simulink subsystem "PvtSubSys_VSM_TSR"  (R2020b)
settings: Solver=VariableStepAuto  StartTime=0.0  StopTime=10.0  RelTol=1e-3
values from neighbouring files (symbols this model uses):
  P_VSM_TSR_Dis_keep_SPL_Table : value not decoded    [TSR.sldd]
  P_VSM_TSR_Dis_keep_SPLend = 50.0    [TSR.sldd]
  P_VSM_TSR_Dis_keep_TS_Table : value not decoded    [TSR.sldd]
  P_VSM_TSR_Ena_SPLSupp_Table : value not decoded    [TSR.sldd]
  P_VSM_TSR_Ena_TS_Table : value not decoded    [TSR.sldd]
  P_VSM_TSR_SLIF_Speed_High = 150.0    [TSR.sldd]
  P_VSM_TSR_SLIF_Speed_Low = 0.0    [TSR.sldd]
  P_VSM_TSR_SLW_SnvtySwitch = 0.0    [TSR.sldd]
  P_VSM_TSR_SLW_Speed_Delta_disable = 1.0    [TSR.sldd]
  P_VSM_TSR_SLW_Speed_Delta_enable = 0.0    [TSR.sldd]
  P_VSM_TSR_SLW_Speed_High = 150.0    [TSR.sldd]
  P_VSM_TSR_SLW_Speed_Low = 30.0    [TSR.sldd]
  P_VSM_TSR_SLW_TrafEyeAvtiveDist = 100.0    [TSR.sldd]
  P_VSM_TSR_SLW_Warning_Time = 10.0    [TSR.sldd]
  P_VSM_TSR_SteerWheelAngle = 360.0    [TSR.sldd]
  P_VSM_TSR_SWS_speed_withDir = 9.0    [TSR.sldd]
  P_VSM_TSR_SWS_speed_woDir = 24.0    [TSR.sldd]
libraries: simulink x23
(part 1 of 2)
settings Model: Creator=GW00133806  LastModifiedBy=GW00201299

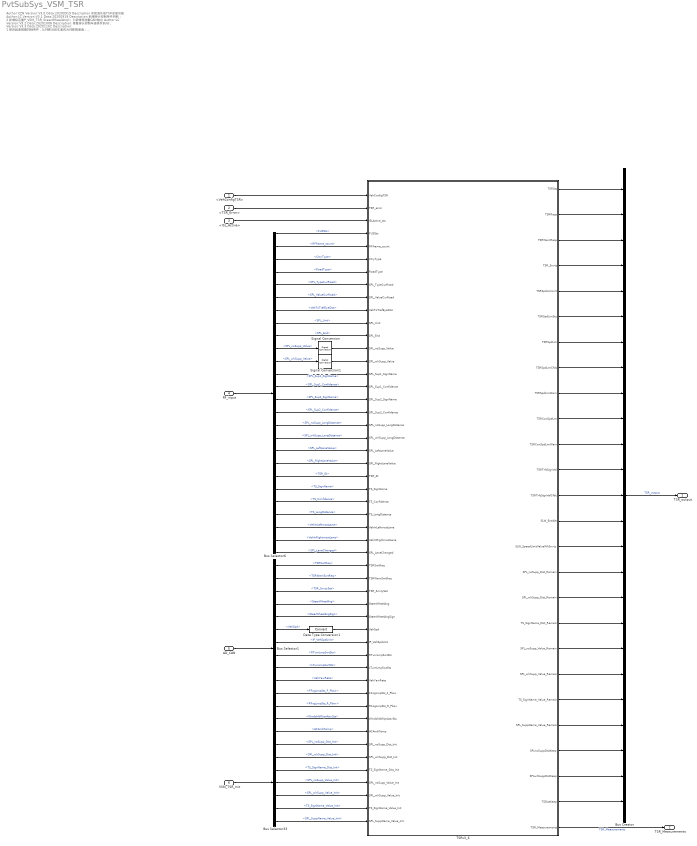
== system PvtSubSys_VSM_TSR ==
  note: Author:CZN
      | Version:V3.0
      | Data:20200919
      | Description:
      | 1.实现海外版TSR全部功能
      | Author:LC
      | Version:V3.1
      | Data:20200919
      | Description:
      | 1.新增掉头抑制条件判断；
      | 2.新增标定量P_VSM_TSR_SteerWheelAngle；
      | 3.新增观测量CAN输出
      | Author:LC
      | Version:V3.2
      | Data:20201008
      | Description:
      | 1.修复掉头抑制车速条件BUG；
      | Version:V3.3
      | Data:20201102
      | Description:
      | 1.修改超速报警抑制条件，从判断当前车速改为判断限速值；
      | 2.修改TSR_error条件下的状态跳转
      | 3.增加了灵敏度设置限幅；
      | 4.更改SLW_Enable信号来源；
      | 5.修复车速单位为英里时，报警值为公里数值问题；
      | 6.更改限速报警限速策略,改为融合发出信息就显示；
      | Version:V3.4
      | Data:20201103
      | Description:
      | 1、新增三个观测量；
      | 2、新增限速使能触发判断；
      | Version:V3.5
      | Data:20201105
      | Description:
      | 1、按照《交通标志信息功能规范》，新增仪表双位灯输出策略；
      | Version:V3.6
      | Data:20201201
      | Description:
      | 1、条件限速使能改为触发式；
      | 20210308
      | 优化转弯限速抑制判断；
      | 20210322
      | 限速条件标志抑制BUG修复；
      | 20210326
      | 1、修复条件限速触发时限速保持距离仍为默认值BUG；
      | 2、修复当超出限速保持距离时，TSR模块将发给仪表的限速清除了，但发给ISL的限速信息漏清BUG；
      | 20210517
      | 修复BUG；当识别到限速标志后3s内不响应解除限速；
      | 20210709:
      | 修复同时识别到限速与接触限速标志后显示解除限速BUG；
  <VehConfigTSR> : Inport
  <TSR_Error> : Inport  Port=2
  <ISL_Active> : Inport  Port=3
  RF_input : Inport  Port=4  OutDataTypeStr=Bus: RFM_TSR_BUS
  AD_CAN : Inport  Port=5  OutDataTypeStr=Bus: AD_TSR_CAN
  VSM_TSR_Init : Inport  Port=6  OutDataTypeStr=Bus: VSM_TSR_INIT_BUS
  Bus Creator : BusCreator  Inputs=25
  Bus Selector1 : BusSelector  OutputSignals=TSRSwtReq,TSRWarnSwtReq,TSR_SnvtySet,SteerWheelAng,SteerWheelAngSign,VehSpd,IP_VehSpdUnit,RTurnLmpSwtSts,LTurnLmpSwtSts,VehYawRate,FFogLmpSts_F_Pbox,RFogLmpSts_R_Pbox,WindshldWiprActvSts,ACAmbTemp
  Bus Selector33 : BusSelector  OutputSignals=SPL_noSupp_Dist_Init,SPL_whSupp_Dist_Init,TS_SignName_Dist_Init,SPL_noSupp_Value_Init,SPL_whSupp_Value_Init,TS_SignName_Value_Init,SPL_SuppName_Value_Init
  Bus Selector6 : BusSelector  OutputSignals=FUSSts,RFframe_count,CtryType,RoadType,SPL_TypeCurRoad,SPL_ValueCurRoad,VehToTrafEyeDist,SPL_Unit,SPL_End,SPL_noSupp_Value,SPL_whSupp_Value,SPL_Sup1_SignName,SPL_Sup1_Confidence,SPL_Sup2_SignName,SPL_Sup2_Confidence,SPL_noSupp_LongDistance,SPL_whSupp_LongDistance,SPL_LeftLaneValue,SPL_RightLaneValue,TSR_ID,TS_SignName,TS_Confidence,TS_LongDistance,VehInLeftmostLane,VehInRightmostLane,SPL_LaneChanged
  Data Type Conversion1 : DataTypeConversion
  Signal Conversion : SignalConversion  OverrideOpt=off
  Signal Conversion1 : SignalConversion  OverrideOpt=off
  TSRv3_6 : Subsystem
  TSR_output : Outport  OutDataTypeStr=Bus: TSR_BUS
  TSR_Measurements : Outport  Port=2  OutDataTypeStr=Bus: VSM_TSR_TSR_Measurements
  wires:
  Signal Conversion/1 -> TSRv3_6/13(SPL_noSupp_Value)
  Bus Selector6/11 -> Signal Conversion1/1  "<SPL_whSupp_Value>"
  Bus Selector33/5 -> TSRv3_6/48(SPL_whSupp_Value_Init)  "<SPL_whSupp_Value_Init>"
  Bus Selector6/26 -> TSRv3_6/29(SPL_LaneChanged)  "<SPL_LaneChanged>"
  Bus Selector1/2 -> TSRv3_6/31(TSRWarnSwtReq)  "<TSRWarnSwtReq>"
  Bus Selector6/16 -> TSRv3_6/19(SPL_noSupp_LongDistance)  "<SPL_noSupp_LongDistance>"
  TSRv3_6/9(TSRSpdLimWarn) -> Bus Creator/9
  Data Type Conversion1/1 -> TSRv3_6/35(VehSpd)
  Bus Selector33/6 -> TSRv3_6/49(TS_SignName_Value_Init)  "<TS_SignName_Value_Init>"
  Bus Selector6/5 -> TSRv3_6/8(SPL_TypeCurRoad)  "<SPL_TypeCurRoad>"
  TSRv3_6/22(SPL_SuppName_Value_Remain) -> Bus Creator/22
  TSRv3_6/1(TSRSts) -> Bus Creator/1
  TSRv3_6/23(SPLnoSuppDistKeep) -> Bus Creator/23
  TSRv3_6/25(TSDistKeep) -> Bus Creator/25
  TSRv3_6/6(TSRSpdLimSts) -> Bus Creator/6
  TSRv3_6/7(TSRSpdLim) -> Bus Creator/7
  Bus Selector33/1 -> TSRv3_6/44(SPL_noSupp_Dist_Init)  "<SPL_noSupp_Dist_Init>"
  Bus Selector6/6 -> TSRv3_6/9(SPL_ValueCurRoad)  "<SPL_ValueCurRoad>"
  Bus Selector6/18 -> TSRv3_6/21(SPL_LeftLaneValue)  "<SPL_LeftLaneValue>"
  Bus Selector6/13 -> TSRv3_6/16(SPL_Sup1_Confidence)  "<SPL_Sup1_Confidence>"
  Bus Selector1/6 -> Data Type Conversion1/1  "<VehSpd>"
  Bus Selector6/24 -> TSRv3_6/27(VehInLeftmostLane)  "<VehInLeftmostLane>"
  TSRv3_6/15(SLW_SpeedLimitValueWhSnvty) -> Bus Creator/15
  TSRv3_6/4(TSR_Snvty) -> Bus Creator/4
  TSRv3_6/10(TSRConSpdLim) -> Bus Creator/10
  TSRv3_6/13(TSRTrfcSignValCfdc) -> Bus Creator/13
  Bus Selector1/11 -> TSRv3_6/40(FFogLmpSts_F_Pbox)  "<FFogLmpSts_F_Pbox>"
  Bus Selector1/8 -> TSRv3_6/37(RTurnLmpSwtSts)  "<RTurnLmpSwtSts>"
  TSRv3_6/26(TSR_Measurements) -> TSR_Measurements/1  "TSR_Measurements"
  TSRv3_6/21(TS_SignName_Value_Remain) -> Bus Creator/21
  Bus Selector6/23 -> TSRv3_6/26(TS_LongDistance)  "<TS_LongDistance>"
  Bus Selector6/22 -> TSRv3_6/25(TS_Confidence)  "<TS_Confidence>"
  Bus Selector6/9 -> TSRv3_6/12(SPL_End)  "<SPL_End>"
  Bus Selector6/14 -> TSRv3_6/17(SPL_Sup2_SignName)  "<SPL_Sup2_SignName>"
  Bus Selector6/8 -> TSRv3_6/11(SPL_Unit)  "<SPL_Unit>"
  Bus Creator/1 -> TSR_output/1  "TSR_output"
  Bus Selector33/4 -> TSRv3_6/47(SPL_noSupp_Value_Init)  "<SPL_noSupp_Value_Init>"
  Bus Selector1/14 -> TSRv3_6/43(ACAmbTemp)  "<ACAmbTemp>"
  Bus Selector1/4 -> TSRv3_6/33(SteerWheelAng)  "<SteerWheelAng>"
  TSRv3_6/24(SPLwhSuppDistKeep) -> Bus Creator/24
  Bus Selector6/2 -> TSRv3_6/5(RFframe_count)  "<RFframe_count>"
  Bus Selector1/10 -> TSRv3_6/39(VehYawRate)  "<VehYawRate>"
  TSRv3_6/14(SLW_Enable) -> Bus Creator/14
  Bus Selector6/1 -> TSRv3_6/4(FUSSts)  "<FUSSts>"
  TSRv3_6/11(TSRConSpdLimWarn) -> Bus Creator/11
  Bus Selector33/2 -> TSRv3_6/45(SPL_whSupp_Dist_Init)  "<SPL_whSupp_Dist_Init>"
  Bus Selector6/4 -> TSRv3_6/7(RoadType)  "<RoadType>"
  TSRv3_6/18(TS_SignName_Dist_Remain) -> Bus Creator/18
  Bus Selector1/3 -> TSRv3_6/32(TSR_SnvtySet)  "<TSR_SnvtySet>"
  TSRv3_6/12(TSRTrfcSignVal) -> Bus Creator/12
  TSRv3_6/19(SPL_noSupp_Value_Remain) -> Bus Creator/19
  Bus Selector1/1 -> TSRv3_6/30(TSRSwtReq)  "<TSRSwtReq>"
  TSRv3_6/8(TSRSpdLimCfdc) -> Bus Creator/8
  Bus Selector6/12 -> TSRv3_6/15(SPL_Sup1_SignName)  "<SPL_Sup1_SignName>"
  TSRv3_6/2(TSRResp) -> Bus Creator/2
  Bus Selector6/21 -> TSRv3_6/24(TS_SignName)  "<TS_SignName>"
  Bus Selector6/19 -> TSRv3_6/22(SPL_RightLaneValue)  "<SPL_RightLaneValue>"
  TSRv3_6/5(TSRSpdLimUnit) -> Bus Creator/5
  Bus Selector6/15 -> TSRv3_6/18(SPL_Sup2_Confidence)  "<SPL_Sup2_Confidence>"
  TSRv3_6/16(SPL_noSupp_Dist_Remain) -> Bus Creator/16
  Bus Selector6/17 -> TSRv3_6/20(SPL_whSupp_LongDistance)  "<SPL_whSupp_LongDistance>"
  Bus Selector1/5 -> TSRv3_6/34(SteerWheelAngSign)  "<SteerWheelAngSign>"
  TSRv3_6/20(SPL_whSupp_Value_Remain) -> Bus Creator/20
  Bus Selector6/10 -> Signal Conversion/1  "<SPL_noSupp_Value>"
  Bus Selector6/3 -> TSRv3_6/6(CtryType)  "<CtryType>"
  Bus Selector33/3 -> TSRv3_6/46(TS_SignName_Dist_Init)  "<TS_SignName_Dist_Init>"
  Bus Selector1/7 -> TSRv3_6/36(IP_VehSpdUnit)  "<IP_VehSpdUnit>"
  <TSR_Error>/1 -> TSRv3_6/2(TSR_error)
  TSRv3_6/17(SPL_whSupp_Dist_Remain) -> Bus Creator/17
  Bus Selector1/12 -> TSRv3_6/41(RFogLmpSts_R_Pbox)  "<RFogLmpSts_R_Pbox>"
  AD_CAN/1 -> Bus Selector1/1
  Bus Selector6/7 -> TSRv3_6/10(VehToTrafEyeDist)  "<VehToTrafEyeDist>"
  Bus Selector1/13 -> TSRv3_6/42(WindshldWiprActvSts)  "<WindshldWiprActvSts>"
  Bus Selector1/9 -> TSRv3_6/38(LTurnLmpSwtSts)  "<LTurnLmpSwtSts>"
  VSM_TSR_Init/1 -> Bus Selector33/1
  RF_input/1 -> Bus Selector6/1
  <ISL_Active>/1 -> TSRv3_6/3(ISLActive_sts)
  Bus Selector6/20 -> TSRv3_6/23(TSR_ID)  "<TSR_ID>"
  Bus Selector33/7 -> TSRv3_6/50(SPL_SuppName_Value_Init)  "<SPL_SuppName_Value_Init>"
  <VehConfigTSR>/1 -> TSRv3_6/1(VehConfigTSR)
  Signal Conversion1/1 -> TSRv3_6/14(SPL_whSupp_Value)
  TSRv3_6/3(TSRWarnResp) -> Bus Creator/3
  Bus Selector6/25 -> TSRv3_6/28(VehInRightmostLane)  "<VehInRightmostLane>"

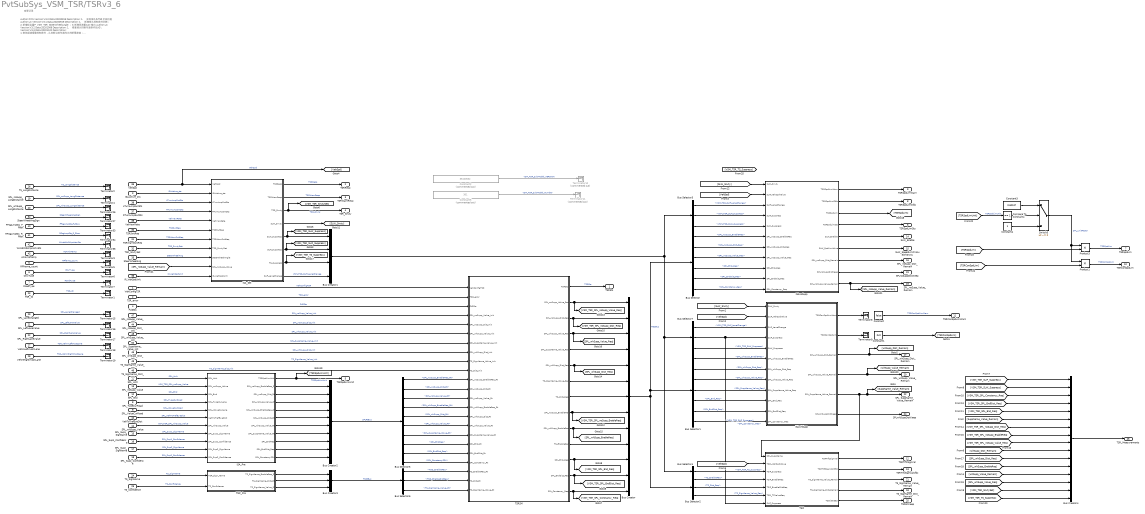
== system PvtSubSys_VSM_TSR/TSRv3_6 ==
  note: 变更记录
  note: Author:CZN
      | Version:V3.0
      | Data:20200919
      | Description:
      | 1.实现海外版TSR全部功能
      | Author:LC
      | Version:V3.1
      | Data:20200919
      | Description:
      | 1.新增掉头抑制条件判断；
      | 2.新增标定量P_VSM_TSR_SteerWheelAngle；
      | 3.新增观测量CAN输出
      | Author:LC
      | Version:V3.2
      | Data:20201008
      | Description:
      | 1.修复掉头抑制车速条件BUG；
      | Version:V3.3
      | Data:20201102
      | Description:
      | 1.修改超速报警抑制条件，从判断当前车速改为判断限速值；
      | 2.修改TSR_error条件下的状态跳转
      | 3.增加了灵敏度设置限幅；
      | 4.更改SLW_Enable信号来源；
      | 5.修复车速单位为英里时，报警值为公里数值问题；
      | 6.更改限速报警限速策略,改为融合发出信息就显示；
      | Version:V3.4
      | Data:20201103
      | Description:
      | 1、新增三个观测量；
      | 2、新增限速使能触发判断；
      | Version:V3.5
      | Data:20201105
      | Description:
      | 1、按照《交通标志信息功能规范》，新增仪表双位灯输出策略；
      | Version:V3.6
      | Data:20201201
      | Description:
      | 1、条件限速使能改为触发式；
      | 20210308
      | 优化转弯限速抑制判断；
      | 20210326
      | 1、修复条件限速触发时限速保持距离仍为默认值BUG；
      | 2、修复当超出限速保持距离时，TSR模块将发给仪表的限速清除了，但发给ISL的限速信息漏清BUG
      | 20210517
      | 修复BUG；当识别到限速标志后3s内不响应解除限速；
  VehConfigTSR : Inport  OutDataTypeStr=uint8
  TSR_error : Inport  Port=2  OutDataTypeStr=uint8
  ISLActive_sts : Inport  Port=3  OutDataTypeStr=boolean
  FUSSts : Inport  Port=4  OutDataTypeStr=uint8
  RFframe_count : Inport  Port=5  OutDataTypeStr=uint32
  CtryType : Inport  Port=6
  RoadType : Inport  Port=7
  SPL_TypeCurRoad : Inport  Port=8  OutDataTypeStr=uint8
  SPL_ValueCurRoad : Inport  Port=9  OutDataTypeStr=uint8
  VehToTrafEyeDist : Inport  Port=10  OutDataTypeStr=uint16
  SPL_Unit : Inport  Port=11  OutDataTypeStr=uint8
  SPL_End : Inport  Port=12  OutDataTypeStr=uint8
  SPL_noSupp_Value : Inport  Port=13  OutDataTypeStr=uint8
  SPL_whSupp_Value : Inport  Port=14  OutDataTypeStr=uint8
  SPL_Sup1_SignName : Inport  Port=15  OutDataTypeStr=uint8
  SPL_Sup1_Confidence : Inport  Port=16  OutDataTypeStr=single
  SPL_Sup2_SignName : Inport  Port=17  OutDataTypeStr=uint8
  SPL_Sup2_Confidence : Inport  Port=18  OutDataTypeStr=single
  SPL_noSupp_LongDistance : Inport  Port=19  OutDataTypeStr=uint8
  SPL_whSupp_LongDistance : Inport  Port=20  OutDataTypeStr=uint8
  SPL_LeftLaneValue : Inport  Port=21  OutDataTypeStr=uint8
  SPL_RightLaneValue : Inport  Port=22  OutDataTypeStr=uint8
  TSR_ID : Inport  Port=23  OutDataTypeStr=uint8
  TS_SignName : Inport  Port=24  OutDataTypeStr=uint8
  TS_Confidence : Inport  Port=25  OutDataTypeStr=single
  TS_LongDistance : Inport  Port=26  OutDataTypeStr=uint8
  VehInLeftmostLane : Inport  Port=27  OutDataTypeStr=uint8
  VehInRightmostLane : Inport  Port=28  OutDataTypeStr=uint8
  SPL_LaneChanged : Inport  Port=29  OutDataTypeStr=uint8
  TSRSwtReq : Inport  Port=30  OutDataTypeStr=boolean
  TSRWarnSwtReq : Inport  Port=31  OutDataTypeStr=boolean
  TSR_SnvtySet : Inport  Port=32  OutDataTypeStr=int8
  SteerWheelAng : Inport  Port=33  OutDataTypeStr=single
  SteerWheelAngSign : Inport  Port=34  OutDataTypeStr=boolean
  VehSpd : Inport  Port=35  OutDataTypeStr=single
  IP_VehSpdUnit : Inport  Port=36  OutDataTypeStr=boolean
  RTurnLmpSwtSts : Inport  Port=37  OutDataTypeStr=boolean
  LTurnLmpSwtSts : Inport  Port=38  OutDataTypeStr=boolean
  VehYawRate : Inport  Port=39  OutDataTypeStr=single
  FFogLmpSts_F_Pbox : Inport  Port=40  OutDataTypeStr=boolean
  RFogLmpSts_R_Pbox : Inport  Port=41  OutDataTypeStr=boolean
  WindshldWiprActvSts : Inport  Port=42  OutDataTypeStr=boolean
  ACAmbTemp : Inport  Port=43  OutDataTypeStr=single
  SPL_noSupp_Dist_Init : Inport  Port=44  OutDataTypeStr=single
  SPL_whSupp_Dist_Init : Inport  Port=45  OutDataTypeStr=single
  TS_SignName_Dist_Init : Inport  Port=46  OutDataTypeStr=single
  SPL_noSupp_Value_Init : Inport  Port=47  OutDataTypeStr=uint8
  SPL_whSupp_Value_Init : Inport  Port=48  OutDataTypeStr=uint8
  TS_SignName_Value_Init : Inport  Port=49  OutDataTypeStr=uint8
  SPL_SuppName_Value_Init : Inport  Port=50  OutDataTypeStr=uint8
  Bus Creator : BusCreator  Inputs=13
  Bus Creator1 : BusCreator  Inputs=4
  Bus Creator2 : BusCreator  Inputs=10
  Bus Creator3 : BusCreator  Inputs=3
  Bus Creator4 : BusCreator  Inputs=16
  Bus Selector : BusSelector  OutputSignals=SPL_noSupp_EnableReq,SPL_noSupp_Dist_Req,SPL_noSupp_Value_Req,SPL_End_Req,SPL_EndDist_Req,SPL_Constancy_Req
  Bus Selector1 : BusSelector  OutputSignals=SPL_whSupp_EnableReq,SPL_whSupp_Dist_Req,SPL_whSupp_Value_Req,SPL_SuppName_Value_Req,SPL_End_Req,SPL_EndDist_Req,SPL_Constancy_Req
  Bus Selector2 : BusSelector  OutputSignals=TS_EnableReq,TS_Dist_Req,TS_SignName_Value_Req
  Bus Selector3 : BusSelector  OutputSignals=VSM_TSR_SLIF_LaneChange,VSM_TSR_SLIF_Suppress,VSM_TSR_SLW_Suppress
  Bus Selector4 : BusSelector  OutputSignals=VSM_TSR_TS_Suppress
  Bus Selector5 : BusSelector  OutputSignals=SPL_noSupp_EnableReq_Rt,SPL_noSupp_Dist_Rt,SPL_noSupp_Value_Rt,SPL_whSupp_EnableReq_Rt,SPL_whSupp_Dist_Rt,SPL_whSupp_Value_Rt,SPL_SuppName_Value_Rt,SPL_EndReq,SPL_EndDist_Req,SPL_ConstancySPL
  Bus Selector6 : BusSelector  OutputSignals=TSD_EnableReq,TSD_EnableDistReq,TS_SignName_Value_Rt
  Bus Selector7 : BusSelector  OutputSignals=VSM_TSR_SLIF_LaneChange,VSM_TSR_SLIF_Suppress,VSM_TSR_SLW_Suppress
  Compare To Constant4 : simulink/Logic and Bit Operations/Compare To Constant  relop===  const=1  OutDataTypeStr=boolean
  Constant : Constant  Value=false  OutDataTypeStr=boolean
  Constant1 : Constant  Value=0x0  OutDataTypeStr=uint8
  Constant2 : Constant  Commented=on  Value=35100532  OutDataTypeStr=uint32
  Constant3 : Constant  Value=0.62137
  Constant4 : Constant
  Constant5 : Constant  Commented=on  Value=301  OutDataTypeStr=uint16
  ISA_Pre : Subsystem
  ISA_Set : Subsystem
  ISAnoSupp : Subsystem
  ISAwhSupp : Subsystem
  Product1 : Product  OutDataTypeStr=uint8
  Product3 : Product  OutDataTypeStr=uint8
  Switch5 : Switch  Criteria=u2 ~= 0  Threshold=1  OutDataTypeStr=single
  TSIF : Subsystem
  TSIF_Pre : Subsystem
  TSRSM : Stateflow chart  TreatAsAtomicUnit=on
  Terminator{1..9,15..19,26..27,33..34,36} (19 alike) : Terminator
  Terminator10 : Terminator  Commented=on
  Terminator11 : Terminator  Commented=on
  TSRSts : Outport
  TSRResp : Outport  Port=2
  TSRWarnResp : Outport  Port=3
  TSR_Snvty : Outport  Port=4  OutDataTypeStr=int8
  TSRSpdLimUnit : Outport  Port=5
  TSRSpdLimSts : Outport  Port=6  OutDataTypeStr=uint8
  TSRSpdLim : Outport  Port=7  OutDataTypeStr=uint8
  TSRSpdLimCfdc : Outport  Port=8  OutDataTypeStr=uint8
  TSRSpdLimWarn : Outport  Port=9  OutDataTypeStr=boolean
  TSRConSpdLim : Outport  Port=10  OutDataTypeStr=uint8
  TSRConSpdLimWarn : Outport  Port=11  OutDataTypeStr=boolean
  TSRTrfcSignVal : Outport  Port=12  OutDataTypeStr=uint8
  TSRTrfcSignValCfdc : Outport  Port=13  OutDataTypeStr=uint8
  SLW_Enable : Outport  Port=14  OutDataTypeStr=boolean
  SLW_SpeedLimitValueWhSnvty : Outport  Port=15  OutDataTypeStr=uint8
  SPL_noSupp_Dist_Remain : Outport  Port=16  OutDataTypeStr=single
  SPL_whSupp_Dist_Remain : Outport  Port=17
  TS_SignName_Dist_Remain : Outport  Port=18  OutDataTypeStr=single
  SPL_noSupp_Value_Remain : Outport  Port=19  OutDataTypeStr=uint8
  SPL_whSupp_Value_Remain : Outport  Port=20  OutDataTypeStr=uint8
  TS_SignName_Value_Remain : Outport  Port=21  OutDataTypeStr=uint8
  SPL_SuppName_Value_Remain : Outport  Port=22  OutDataTypeStr=uint8
  SPLnoSuppDistKeep : Outport  Port=23  OutDataTypeStr=single
  SPLwhSuppDistKeep : Outport  Port=24  OutDataTypeStr=single
  TSDistKeep : Outport  Port=25
  TSR_Measurements : Outport  Port=26
  wires:
  Constant5/1 -> Terminator11/1  "VSM_TSR_SubModel_Number"
  Constant2/1 -> Terminator10/1  "VSM_TSR_SubModel_VERSION"
  ISA_Set/2(TSRWarnResp) -> TSRWarnResp/1  "TSRWarnResp"
  SPL_noSupp_LongDistance/1 -> Terminator4/1  "SPL_noSupp_LongDistance"
  FFogLmpSts_F_Pbox/1 -> Terminator33/1  "FFogLmpSts_F_Pbox"
  ISA_Set/8(SLIF_LaneChange) -> Bus Creator1/4  "VSM_TSR_SLIF_LaneChange"
  ISAnoSupp/3(TSRSpdLim) -> [TSRSpdLim]
  FUSSts/1 -> TSRSM/3(FUSSts)  "FUSSts"
  ISAnoSupp/7(SPL_noSupp_Dist_Remain) -> SPL_noSupp_Dist_Remain/1
  VehConfigTSR/1 -> TSRSM/1(VehConfigTSR)  "VehConfigTSR"
  SPL_noSupp_Value/1 -> ISA_Pre/2(SPL_noSupp_Value)  "VSM_TSR_SPL_noSupp_Value"
  Bus Selector/4 -> ISAnoSupp/9(SPL_End_Req)  "<SPL_End_Req>"
  WindshldWiprActvSts/1 -> Terminator36/1  "WindshldWiprActvSts"
  [VehSpd] -> ISAnoSupp/2(SLIF_VehSpdValue)
  RTurnLmpSwtSts/1 -> ISA_Set/4(RTurnLmpSwtSts)  "RTurnLmpSwtSts"
  ISLActive_sts/1 -> ISA_Set/2(ISLActive_sts)  "ISLActive_sts"
  ISAnoSupp/8(SPLnoSuppDistKeep) -> SPLnoSuppDistKeep/1
  Bus Selector/5 -> ISAnoSupp/10(SPL_EndDist_Req)  "<SPL_EndDist_Req>"
  SPL_ValueCurRoad/1 -> ISA_Pre/5(SPL_ValueCurLane)  "SPL_ValueCurRoad"
  ISA_Set/1(TSRResp) -> TSRResp/1  "TSRResp"
  CtryType/1 -> Terminator6/1  "CtryType"
  TSRWarnSwtReq/1 -> ISA_Set/7(TSRWarnSwtReq)  "TSRWarnSwtReq"
  SteerWheelAngSign/1 -> Terminator27/1  "SteerWheelAngSign"
  VehToTrafEyeDist/1 -> ISA_Pre/6(VehToTrafEyeDist)  "SPL_VehToTrafEyeDist"
  ISA_Set/5(SLW_Suppress) -> Bus Creator1/1, [VSM_TSR_SLW_Suppress]
  TS_SignName/1 -> TSIF_Pre/1(TSR_Sign_Name)  "TS_SignName"
  TSRSwtReq/1 -> ISA_Set/6(TSRSwtReq)  "TSRSwtReq"
  TSIF/3(TS_SignName_Value_Remain) -> TS_SignName_Value_Remain/1
  TSIF/1(TSRTrfcSignVal) -> TSRTrfcSignVal/1
  SPL_whSupp_LongDistance/1 -> Terminator26/1  "SPL_whSupp_LongDistance"
  RFframe_count/1 -> Terminator5/1  "RFframe_count"
  SPL_End/1 -> ISA_Pre/3(SPL_End)  "SPL_End"
  TSRSM/1(TSRSts) -> TSRSts/1  "TSRSts"
  ISAwhSupp/5(SPL_SuppName_Value_Remain) -> TSIF/1(SPL_SuppName), [SuppName_Value_Remain], SPL_SuppName_Value_Remain/1
  SPL_LeftLaneValue/1 -> Terminator16/1  "SPL_LeftLaneValue"
  [SLW_Snvty] -> ISAnoSupp/1(SLW_Snvty)
  SteerWheelAng/1 -> ISA_Set/9(SteerWheelAngle)  "SteerWheelAng"
  ISAnoSupp/6(SLW_SpdLimValue) -> SLW_SpeedLimitValueWhSnvty/1
  SPL_LaneChanged/1 -> Terminator15/1  "SPL_LaneChanged"
  VehInRightmostLane/1 -> Terminator19/1  "TSR_VehInRightmostLane"
  SPL_SuppName_Value_Init/1 -> TSRSM/7(SPL_SuppName_Value_Init)  "SPL_SuppName_Value_Init"
  [VehSpd] -> TSIF/2(TSD_VehSpdValue)
  SPL_whSupp_Value/1 -> ISA_Pre/7(SPL_whSupp_Value)  "VSM_TSR_SPL_whSupp_Value"
  RFogLmpSts_R_Pbox/1 -> Terminator34/1  "RFogLmpSts_R_Pbox"
  SPL_whSupp_Value_Init/1 -> TSRSM/6(SPL_whSupp_Value_Init)  "SPL_whSupp_Value_Init"
  ISAnoSupp/4(TSRSpdLimSts) -> TSRSpdLimSts/1
  SPL_noSupp_Dist_Init/1 -> TSRSM/5(SPL_noSupp_Dist_Init)  "SPL_noSupp_Dist_Init"
  LTurnLmpSwtSts/1 -> ISA_Set/3(LTurnLmpSwtSts)  "LTurnLmpSwtSts"
  VehYawRate/1 -> ISA_Set/5(VehYawRate)  "VehYawRate"
  SPL_whSupp_Dist_Init/1 -> TSRSM/8(SPL_whSupp_Dist_Init)  "SPL_whSupp_Dist_Init"
  VehInLeftmostLane/1 -> Terminator18/1  "TSR_VehInLeftmostLane"
  TSR_error/1 -> TSRSM/2(TSR_error)  "TSR_error"
  Bus Selector/6 -> ISAnoSupp/11(SPL_Constancy_Req)  "<SPL_Constancy_Req>"
  TSIF/2(TSRTrfcSignValCfdc) -> TSRTrfcSignValCfdc/1
  TS_SignName_Dist_Init/1 -> TSRSM/10(TS_Dist_Init)  "TS_SignName_Dist_Init"
  Bus Selector3/1 -> ISAnoSupp/3(SLIF_LaneChange)  "<VSM_TSR_SLIF_LaneChange>"
  TS_SignName_Value_Init/1 -> TSRSM/9(TS_SignName_Value_Init)  "TS_SignName_Value_Init"
  SPL_RightLaneValue/1 -> Terminator17/1  "SPL_RightLaneValue"
  TS_LongDistance/1 -> Terminator2/1  "TS_LongDistance"
  ISA_Set/6(SLIF_Suppress) -> Bus Creator1/2, [VSM_TSR_SLIF_Suppress]
  ISAwhSupp/4(SPL_whSupp_Value_Remain) -> [whSupp_Value_Remain], SPL_whSupp_Value_Remain/1
  TSIF/4(TS_SignName_Dist_Remain) -> TS_SignName_Dist_Remain/1
  SPL_TypeCurRoad/1 -> ISA_Pre/4(SPL_TypeCurLane)  "SPL_TypeCurRoad"
  SPL_noSupp_Value_Init/1 -> TSRSM/4(SPL_noSupp_Value_Init)  "SPL_noSupp_Value_Init"
  VehSpd/1 -> [VehSpd], ISA_Set/1(VehSpd)  "VehSpd"
  ISAwhSupp/3(SPL_whSupp_Dist_Remain) -> [whSupp_Dist_Remain], SPL_whSupp_Dist_Remain/1
  ACAmbTemp/1 -> Terminator3/1  "ACAmbTemp"
  RoadType/1 -> Terminator7/1  "RoadType"
  TS_Confidence/1 -> TSIF_Pre/2(TS_Confidence)  "TS_Confidence"
  TSR_ID/1 -> Terminator1/1  "TSR_ID"
  ISAwhSupp/1(TSRConSpdLimWarn) -> Terminator8/1
  ISAwhSupp/2(TSRConSpdLim) -> Terminator9/1
  TSIF_Pre/1(TS_SignName_EnableReq_Rt) -> Bus Creator3/1
  TSIF_Pre/2(TS_SignName_Dist_Rt) -> Bus Creator3/2
  TSIF_Pre/3(TS_SignName_Value_Rt) -> Bus Creator3/3
  SPL_Sup1_SignName/1 -> ISA_Pre/8(SPL_Sup1_SignName)  "SPL_Sup1_SignName"
  SPL_Sup1_Confidence/1 -> ISA_Pre/9(SPL_Sup1_Confidence)  "SPL_Sup1_Confidence"
  SPL_Sup2_SignName/1 -> ISA_Pre/10(SPL_Sup2_SignName)  "SPL_Sup2_SignName"
  SPL_Sup2_Confidence/1 -> ISA_Pre/11(SPL_Sup2_Confidence)  "SPL_Sup2_Confidence"
  ISA_Set/7(TS_Suppress) -> Bus Creator1/3, [VSM_TSR_TS_Suppress]
  Bus Selector2/2 -> TSIF/5(TSIF_EnableDistReq)  "<TS_Dist_Req>"
  Bus Selector2/1 -> TSIF/4(TSIF_EnableReq)  "<TS_EnableReq>"
  Bus Selector4/1 -> TSIF/3(TSIF_Suppress)  "<VSM_TSR_TS_Suppress>"
  ISAnoSupp/5(SLW_Enable) -> SLW_Enable/1
  TSRSM/3(SPL_noSupp_Dist_Req) -> [VSM_TSR_SPL_noSupp_Dist_Req], Bus Creator/2
  TSRSM/2(SPL_noSupp_Value_Req) -> [VSM_TSR_SPL_noSupp_Value_Req], Bus Creator/1
  TSRSM/4(SPL_whSupp_Value_Req) -> [SPL_whSupp_Value_Req], Bus Creator/3
  TSRSM/5(SPL_SuppName_Value_Req) -> Bus Creator/4
  TSRSM/6(SPL_whSupp_Dist_Req) -> [SPL_whSupp_Dist_Req], Bus Creator/5
  TSRSM/7(TS_SignName_Value_Req) -> Bus Creator/6
  TSRSM/8(TS_Dist_Req) -> Bus Creator/7
  TSRSM/9(SPL_noSupp_EnableReq) -> [VSM_TSR_SPL_noSupp_EnableReq], Bus Creator/8
  TSRSM/10(SPL_whSupp_EnableReq) -> [SPL_whSupp_EnableReq], Bus Creator/9
  TSRSM/11(TS_EnableReq) -> Bus Creator/10
  Bus Creator/1 -> Bus Selector2/1, Bus Selector/1, Bus Selector1/1  "ReqBus"
  Bus Selector/1 -> ISAnoSupp/6(SPL_noSupp_EnableReq)  "<SPL_noSupp_EnableReq>"
  Bus Selector2/3 -> TSIF/6(TSD_TSValueReq)  "<TS_SignName_Value_Req>"
  Bus Creator1/1 -> Bus Selector7/1, Bus Selector4/1, Bus Selector3/1
  Bus Selector3/2 -> ISAnoSupp/4(SLIF_Suppress)  "<VSM_TSR_SLIF_Suppress>"
  Bus Selector3/3 -> ISAnoSupp/5(SLW_Suppress)  "<VSM_TSR_SLW_Suppress>"
  ISAnoSupp/1(TSRSpdLimWarn) -> TSRSpdLimWarn/1
  Bus Creator2/1 -> Bus Selector5/1  "SPLRtBus"
  ISA_Pre/2(SPL_noSupp_EnableReq_Rt) -> Bus Creator2/1
  ISA_Pre/3(SPL_noSupp_Dist_Rt) -> Bus Creator2/2
  ISA_Pre/4(SPL_noSupp_Value_Rt) -> Bus Creator2/3
  ISA_Pre/5(SPL_whSupp_EnableReq_Rt) -> Bus Creator2/4
  ISA_Pre/6(SPL_whSupp_Dist_Rt) -> Bus Creator2/5
  ISA_Pre/7(SPL_whSupp_Value_Rt) -> Bus Creator2/6
  ISA_Pre/8(SPL_SuppName_Value_Rt) -> Bus Creator2/7
  ISA_Pre/9(SPL_EndReq) -> Bus Creator2/8
  ISA_Pre/10(SPL_EndDist_Req) -> Bus Creator2/9
  ISA_Pre/11(SPL_ConstancySPL) -> Bus Creator2/10
  Bus Selector5/2 -> TSRSM/12(SPL_noSupp_Dist_Rt)  "<SPL_noSupp_Dist_Rt>"
  Bus Selector5/1 -> TSRSM/11(SPL_noSupp_EnableReq_Rt)  "<SPL_noSupp_EnableReq_Rt>"
  Bus Selector5/3 -> TSRSM/13(SPL_noSupp_Value_Rt)  "<SPL_noSupp_Value_Rt>"
  Bus Selector5/4 -> TSRSM/14(SPL_whSupp_EnableReq_Rt)  "<SPL_whSupp_EnableReq_Rt>"
  Bus Selector5/5 -> TSRSM/15(SPL_whSupp_Dist_Rt)  "<SPL_whSupp_Dist_Rt>"
  Bus Selector5/6 -> TSRSM/16(SPL_whSupp_Value_Rt)  "<SPL_whSupp_Value_Rt>"
  Bus Selector5/7 -> TSRSM/17(SPL_SuppName_Value_Rt)  "<SPL_SuppName_Value_Rt>"
  Bus Creator3/1 -> Bus Selector6/1  "TSRtBus"
  Bus Selector6/1 -> TSRSM/21(TS_EnableReq_Rt)  "<TSD_EnableReq>"
  Bus Selector6/2 -> TSRSM/22(TS_Dist_Rt)  "<TSD_EnableDistReq>"
  Bus Selector6/3 -> TSRSM/23(TS_SignName_Value_Rt)  "<TS_SignName_Value_Rt>"
  Bus Selector5/8 -> TSRSM/18(SPL_End_Rt)  "<SPL_EndReq>"
  Bus Selector5/9 -> TSRSM/19(SPL_EndDist_Rt)  "<SPL_EndDist_Req>"
  TSRSM/12(SPL_End_Req) -> [VSM_TSR_SPL_End_Req], Bus Creator/11
  TSRSM/13(SPL_EndDist_Req) -> [VSM_TSR_SPL_EndDist_Req], Bus Creator/12
  TSRSM/14(SPL_Constancy_Req) -> [VSM_TSR_SPL_Constancy_Req], Bus Creator/13
  SPL_Unit/1 -> ISA_Pre/1(SPL_Unit)  "SPL_Unit"
  TSR_SnvtySet/1 -> ISA_Set/8(TSR_SnvtySet)  "TSR_SnvtySet"
  IP_VehSpdUnit/1 -> ISA_Set/11(IP_VehSpdUnit)  "IP_VehSpdUnit"
  ISA_Pre/1(TSRSpdLimUnit) -> [TSRSpdLimUnit], TSRSpdLimUnit/1  "TSRSpdLimUnit"
  ISA_Set/3(TSR_Snvty) -> TSR_Snvty/1, [VSM_TSR_SnvtySet]  "TSR_Snvty"
  ISA_Set/4(SLW_Snvty) -> [SLW_Snvty]
  Bus Selector1/1 -> ISAwhSupp/6(SPL_whSupp_EnableReq)  "<SPL_whSupp_EnableReq>"
  Bus Selector1/2 -> ISAwhSupp/7(SPL_whSupp_Dist_Req)  "<SPL_whSupp_Dist_Req>"
  Bus Selector1/3 -> ISAwhSupp/8(SPL_whSupp_Value_Req)  "<SPL_whSupp_Value_Req>"
  Bus Selector1/4 -> ISAwhSupp/9(SPL_SuppName_Value_Req)  "<SPL_SuppName_Value_Req>"
  Bus Selector7/3 -> ISAwhSupp/5(SLW_Suppress)  "<VSM_TSR_SLW_Suppress>"
  Bus Selector7/2 -> ISAwhSupp/4(SLIF_Suppress), TSIF/7(SLIF_Suppress)  "<VSM_TSR_SLIF_Suppress>"
  Bus Selector7/1 -> ISAwhSupp/3(SLIF_LaneChange)  "<VSM_TSR_SLIF_LaneChange>"
  [SLW_Snvty] -> ISAwhSupp/1(SLW_Snvty)
  [VehSpd] -> ISAwhSupp/2(SLIF_VehSpdValue)
  Bus Selector/2 -> ISAnoSupp/7(SPL_noSupp_Dist_Req)  "<SPL_noSupp_Dist_Req>"
  Bus Selector/3 -> ISAnoSupp/8(SPL_noSupp_Value_Req)  "<SPL_noSupp_Value_Req>"
  Bus Selector5/10 -> TSRSM/20(SPL_Constancy_Rt)  "<SPL_ConstancySPL>"
  ISAwhSupp/6(SPLwhSuppDistKeep) -> SPLwhSuppDistKeep/1
  TSIF/5(TSDistKeep) -> TSDistKeep/1
  Bus Creator4/1 -> TSR_Measurements/1
  [VSM_TSR_SPL_noSupp_Dist_Req] -> Bus Creator4/7
  [VSM_TSR_SPL_noSupp_EnableReq] -> Bus Creator4/8
  [SuppName_Value_Remain] -> Bus Creator4/6
  [VSM_TSR_SPL_noSupp_Value_Req] -> Bus Creator4/9
  [VSM_TSR_SPL_EndDist_Req] -> Bus Creator4/4
  [VSM_TSR_SPL_End_Req] -> Bus Creator4/5
  [VSM_TSR_SPL_Constancy_Req] -> Bus Creator4/3
  [VSM_TSR_SLW_Suppress] -> Bus Creator4/2
  [VSM_TSR_SLIF_Suppress] -> Bus Creator4/1
  [whSupp_Dist_Remain] -> Bus Creator4/10
  [SPL_whSupp_Dist_Req] -> Bus Creator4/11
  [SPL_whSupp_EnableReq] -> Bus Creator4/12
  [whSupp_Value_Remain] -> Bus Creator4/13
  [SPL_whSupp_Value_Req] -> Bus Creator4/14
  [VSM_TSR_SnvtySet] -> Bus Creator4/15
  [VSM_TSR_TS_Suppress] -> Bus Creator4/16
  ISAnoSupp/2(TSRSpdLimCfdc) -> TSRSpdLimCfdc/1
  [SPL_noSupp_Value_Remain] -> ISA_Set/10(SPL_noSupp_Value)
  ISAnoSupp/9(SPL_noSupp_Value_Remain) -> SPL_noSupp_Value_Remain/1, [SPL_noSupp_Value_Remain]
  Constant4/1 -> Switch5/3
  Constant3/1 -> Switch5/1
  [TSRSpdLimUnit] -> Compare To Constant4/1  "TSRSpdLimUnit"
  Compare To Constant4/1 -> Switch5/2
  Switch5/1 -> Product1/1, Product3/1  "SPL_unitFactor"
  [TSRSpdLim] -> Product3/2
  Product3/1 -> TSRSpdLim/1  "TSRSpdLim"
  [TSRConSpdLim] -> Product1/2
  Product1/1 -> TSRConSpdLim/1  "TSRConSpdLim"
  Bus Selector1/5 -> ISAwhSupp/10(SPL_End_Req)  "<SPL_End_Req>"
  Bus Selector1/6 -> ISAwhSupp/11(SPL_EndDist_Req)  "<SPL_EndDist_Req>"
  Bus Selector1/7 -> ISAwhSupp/12(SPL_Constancy_Req)  "<SPL_Constancy_Req>"
  Constant/1 -> TSRConSpdLimWarn/1  "TSRConSpdLimWarn"
  Constant1/1 -> [TSRConSpdLim]

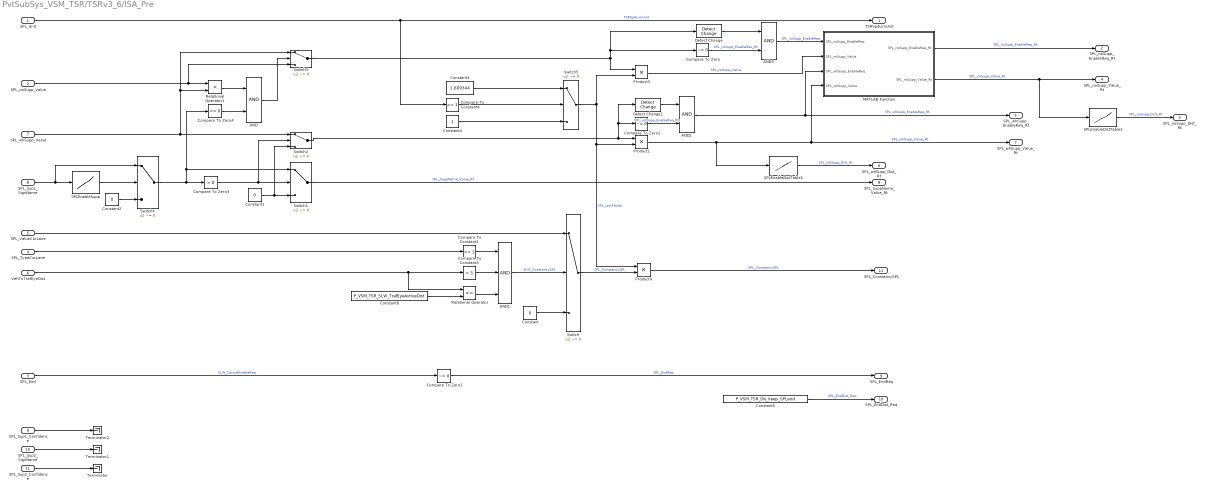
== system PvtSubSys_VSM_TSR/TSRv3_6/ISA_Pre ==
  SPL_Unit : Inport  OutDataTypeStr=uint8
  SPL_noSupp_Value : Inport  Port=2  OutDataTypeStr=uint8
  SPL_End : Inport  Port=3  OutDataTypeStr=uint8
  SPL_TypeCurLane : Inport  Port=4  OutDataTypeStr=uint8
  SPL_ValueCurLane : Inport  Port=5  OutDataTypeStr=uint8
  VehToTrafEyeDist : Inport  Port=6  OutDataTypeStr=uint16
  SPL_whSupp_Value : Inport  Port=7
  SPL_Sup1_SignName : Inport  Port=8  OutDataTypeStr=uint8
  SPL_Sup1_Confidence : Inport  Port=9  OutDataTypeStr=single
  SPL_Sup2_SignName : Inport  Port=10  OutDataTypeStr=uint8
  SPL_Sup2_Confidence : Inport  Port=11  OutDataTypeStr=single
  AND : Logic  AllPortsSameDT=off  OutDataTypeStr=boolean
  AND1 : Logic  Inputs=3  AllPortsSameDT=off  OutDataTypeStr=boolean
  AND2 : Logic  AllPortsSameDT=off  OutDataTypeStr=boolean
  AND3 : Logic  AllPortsSameDT=off  OutDataTypeStr=boolean
  Compare To Constant1 : simulink/Logic and Bit Operations/Compare To Constant  relop===  const=1  OutDataTypeStr=boolean
  Compare To Constant3 : simulink/Logic and Bit Operations/Compare To Constant  relop=>  const=5  OutDataTypeStr=boolean
  Compare To Constant4 : simulink/Logic and Bit Operations/Compare To Constant  relop===  const=1  OutDataTypeStr=boolean
  Compare To Zero : simulink/Logic and Bit Operations/Compare To Zero  relop=~=  OutDataTypeStr=boolean
  Compare To Zero1 : simulink/Logic and Bit Operations/Compare To Zero  relop=~=  OutDataTypeStr=boolean
  Compare To Zero2 : simulink/Logic and Bit Operations/Compare To Zero  relop=~=  OutDataTypeStr=boolean
  Compare To Zero3 : simulink/Logic and Bit Operations/Compare To Zero  relop=>  OutDataTypeStr=boolean
  Compare To Zero4 : simulink/Logic and Bit Operations/Compare To Zero  relop===  OutDataTypeStr=boolean
  Constant : Constant  Value=0  OutDataTypeStr=uint8
  Constant1 : Constant  Value=0  OutDataTypeStr=Inherit: Inherit via back propagation
  Constant2 : Constant  Value=0  OutDataTypeStr=Inherit: Inherit via back propagation
  Constant3 : Constant  Value=1.609344
  Constant4 : Constant
  Constant5 : Constant  Value=P_VSM_TSR_Dis_keep_SPLend  OutDataTypeStr=single
  Constant8 : Constant  Value=P_VSM_TSR_SLW_TrafEyeAvtiveDist
  Detect Change : simulink/Logic and Bit Operations/Detect Change  vinit=0  OutDataTypeStr=boolean
  Detect Change1 : simulink/Logic and Bit Operations/Detect Change  vinit=0  OutDataTypeStr=boolean
  MATLAB Function : MATLAB Function  TreatAsAtomicUnit=on
  Product1 : Product  OutDataTypeStr=uint8
  Product3 : Product  OutDataTypeStr=uint8
  Product4 : Product  OutDataTypeStr=uint8
  Relational Operator : RelationalOperator  Operator=<=  OutDataTypeStr=boolean  RndMeth=Simplest
  Relational Operator1 : RelationalOperator  Operator=<  OutDataTypeStr=boolean  RndMeth=Simplest
  SPLEnableDistTable1 : Lookup_n-D  NumberOfTableDimensions=1  BreakpointsForDimension1=[0:10:150]  BreakpointsForDimension1DataTypeStr=uint8  Table=P_VSM_TSR_Dis_keep_SPL_Table  TableDataTypeStr=Inherit: Inherit from 'Table data'  InterpMethod=Flat  ExtrapMethod=Cubic spline  InternalRulePriority=Speed  OutDataTypeStr=single  RndMeth=Simplest  InputSameDT=on
  SPLEnableDistTable2 : Lookup_n-D  NumberOfTableDimensions=1  BreakpointsForDimension1=[0:10:150]  BreakpointsForDimension1DataTypeStr=uint8  Table=P_VSM_TSR_Dis_keep_SPL_Table  TableDataTypeStr=Inherit: Inherit from 'Table data'  InterpMethod=Flat  ExtrapMethod=Cubic spline  InternalRulePriority=Speed  OutDataTypeStr=single  RndMeth=Simplest  InputSameDT=on
  SPLEnableSupp : Lookup_n-D  NumberOfTableDimensions=1  BreakpointsForDimension1=[0:1:0x16]  BreakpointsForDimension1DataTypeStr=uint8  Table=P_VSM_TSR_Ena_SPLSupp_Table  TableDataTypeStr=Inherit: Inherit from 'Table data'  InterpMethod=Flat  ExtrapMethod=Cubic spline  InternalRulePriority=Speed  OutDataTypeStr=Inherit: Inherit via back propagation  RndMeth=Simplest  InputSameDT=on
  Switch : Switch  Criteria=u2 ~= 0  OutDataTypeStr=uint8
  Switch{1..4} (4 alike) : Switch  Criteria=u2 ~= 0
  Switch5 : Switch  Criteria=u2 ~= 0  Threshold=1  OutDataTypeStr=single
  Terminator : Terminator
  Terminator1 : Terminator
  Terminator2 : Terminator
  TSRSpdLimUnit : Outport  OutDataTypeStr=uint8
  SPL_noSupp_EnableReq_Rt : Outport  Port=2  OutDataTypeStr=boolean
  SPL_noSupp_Dist_Rt : Outport  Port=3  OutDataTypeStr=single
  SPL_noSupp_Value_Rt : Outport  Port=4  OutDataTypeStr=uint8
  SPL_whSupp_EnableReq_Rt : Outport  Port=5  OutDataTypeStr=boolean
  SPL_whSupp_Dist_Rt : Outport  Port=6  OutDataTypeStr=single
  SPL_whSupp_Value_Rt : Outport  Port=7  OutDataTypeStr=uint8
  SPL_SuppName_Value_Rt : Outport  Port=8
  SPL_EndReq : Outport  Port=9  OutDataTypeStr=boolean
  SPL_EndDist_Req : Outport  Port=10  OutDataTypeStr=single
  SPL_ConstancySPL : Outport  Port=11  OutDataTypeStr=uint8
  wires:
  Compare To Zero1/1 -> SPL_EndReq/1  "SPL_EndReq"
  Switch3/1 -> Detect Change/1, Compare To Zero/1, Product3/1
  AND3/1 -> MATLAB Function/1(SPL_noSupp_EnableReq)  "SPL_noSupp_EnableReq"
  Compare To Constant3/1 -> AND1/2
  AND1/1 -> Switch/2  "SLW_ConstancySPL"
  SPL_ValueCurLane/1 -> Switch/1
  SPL_TypeCurLane/1 -> Compare To Constant1/1
  Product3/1 -> MATLAB Function/2(SPL_noSupp_Value)  "SPL_noSupp_Value"
  Relational Operator/1 -> AND1/3
  Constant8/1 -> Relational Operator/2
  SPLEnableDistTable2/1 -> SPL_noSupp_Dist_Rt/1  "SPL_noSupp_Dist_Rt"
  Constant5/1 -> SPL_EndDist_Req/1  "SPL_EndDist_Req"
  SPL_End/1 -> Compare To Zero1/1  "SLW_CancelEnableReq"
  VehToTrafEyeDist/1 -> Relational Operator/1, Compare To Constant3/1
  Compare To Constant1/1 -> AND1/1
  Switch4/1 -> Compare To Zero4/1, Switch1/1, Compare To Zero3/1
  SPLEnableDistTable1/1 -> SPL_whSupp_Dist_Rt/1  "SPL_whSupp_Dist_Rt"
  SPL_Sup2_Confidence/1 -> Terminator/1
  SPL_Sup1_Confidence/1 -> Terminator2/1
  SPL_Sup2_SignName/1 -> Terminator1/1
  Switch2/1 -> Product1/1, Detect Change1/1, Compare To Zero2/1
  Product1/1 -> SPLEnableDistTable1/1, SPL_whSupp_Value_Rt/1, MATLAB Function/4(SPL_whSupp_Value)  "SPL_whSupp_Value_Rt"
  AND2/1 -> SPL_whSupp_EnableReq_Rt/1, MATLAB Function/3(SPL_whSupp_EnableReq)  "SPL_whSupp_EnableReq_Rt"
  Compare To Constant4/1 -> Switch5/2
  SPL_Unit/1 -> Compare To Constant4/1, TSRSpdLimUnit/1  "TSRSpdLimUnit"
  Constant3/1 -> Switch5/1
  Constant4/1 -> Switch5/3
  Switch5/1 -> Product1/2, Product4/1, Product3/2  "SPL_unitFactor"
  Constant/1 -> Switch/3
  Switch/1 -> Product4/2  "SPL_ConstancySPL"
  Product4/1 -> SPL_ConstancySPL/1  "SPL_ConstancySPL"
  Compare To Zero3/1 -> Switch2/2, Switch1/2
  SPL_whSupp_Value/1 -> Switch2/1, Switch3/1, Relational Operator1/2
  Switch1/1 -> SPL_SuppName_Value_Rt/1  "SPL_SuppName_Value_Rt"
  Constant1/1 -> Switch2/3, Switch1/3
  SPL_noSupp_Value/1 -> Switch3/3, Relational Operator1/1
  Relational Operator1/1 -> AND/1
  Compare To Zero4/1 -> AND/2
  AND/1 -> Switch3/2
  SPL_Sup1_SignName/1 -> Switch4/1, SPLEnableSupp/1
  SPLEnableSupp/1 -> Switch4/2
  Constant2/1 -> Switch4/3
  Detect Change/1 -> AND3/1
  Compare To Zero/1 -> AND3/2  "SPL_noSupp_EnableReq_Rt"
  MATLAB Function/2(SPL_noSupp_Value_Rt) -> SPLEnableDistTable2/1, SPL_noSupp_Value_Rt/1  "SPL_noSupp_Value_Rt"
  MATLAB Function/1(SPL_noSupp_EnableReq_Rt) -> SPL_noSupp_EnableReq_Rt/1  "SPL_noSupp_EnableReq_Rt"
  Detect Change1/1 -> AND2/1
  Compare To Zero2/1 -> AND2/2  "SPL_whSupp_EnableReq_Rt"

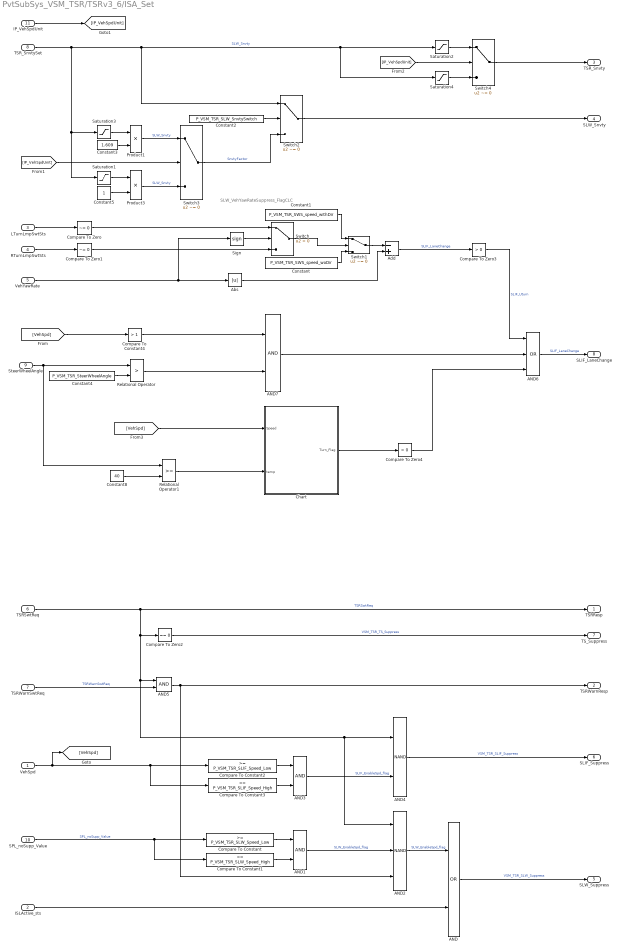
== system PvtSubSys_VSM_TSR/TSRv3_6/ISA_Set ==
  note: SLW_VehYawRateSuppress_FlagCLC
  VehSpd : Inport  OutDataTypeStr=single
  ISLActive_sts : Inport  Port=2  OutDataTypeStr=boolean
  LTurnLmpSwtSts : Inport  Port=3  OutDataTypeStr=boolean
  RTurnLmpSwtSts : Inport  Port=4  OutDataTypeStr=boolean
  VehYawRate : Inport  Port=5  OutDataTypeStr=single
  TSRSwtReq : Inport  Port=6
  TSRWarnSwtReq : Inport  Port=7
  TSR_SnvtySet : Inport  Port=8
  SteerWheelAngle : Inport  Port=9  OutDataTypeStr=single
  SPL_noSupp_Value : Inport  Port=10  OutDataTypeStr=uint8
  IP_VehSpdUnit : Inport  Port=11  OutDataTypeStr=boolean
  AND : Logic  Operator=OR  AllPortsSameDT=off  OutDataTypeStr=boolean
  AND{1,3,5,7} (4 alike) : Logic  AllPortsSameDT=off  OutDataTypeStr=boolean
  AND2 : Logic  Operator=NAND  Inputs=3  AllPortsSameDT=off  OutDataTypeStr=boolean
  AND4 : Logic  Operator=NAND  AllPortsSameDT=off  OutDataTypeStr=boolean
  AND6 : Logic  Operator=OR  Inputs=3  AllPortsSameDT=off  OutDataTypeStr=boolean
  Abs : Abs
  Add : Sum  Inputs=-+
  Chart : Stateflow chart  TreatAsAtomicUnit=on
  Compare To Constant : simulink/Logic and Bit Operations/Compare To Constant  relop=>=  const=P_VSM_TSR_SLW_Speed_Low  OutDataTypeStr=boolean
  Compare To Constant1 : simulink/Logic and Bit Operations/Compare To Constant  relop=<=  const=P_VSM_TSR_SLW_Speed_High  OutDataTypeStr=boolean
  Compare To Constant2 : simulink/Logic and Bit Operations/Compare To Constant  relop=>=  const=P_VSM_TSR_SLIF_Speed_Low  OutDataTypeStr=boolean
  Compare To Constant3 : simulink/Logic and Bit Operations/Compare To Constant  relop=<=  const=P_VSM_TSR_SLIF_Speed_High  OutDataTypeStr=boolean
  Compare To Constant4 : simulink/Logic and Bit Operations/Compare To Constant  relop=>  const=1  OutDataTypeStr=boolean
  Compare To Zero : simulink/Logic and Bit Operations/Compare To Zero  relop=~=  OutDataTypeStr=boolean
  Compare To Zero1 : simulink/Logic and Bit Operations/Compare To Zero  relop=~=  OutDataTypeStr=boolean
  Compare To Zero2 : simulink/Logic and Bit Operations/Compare To Zero  relop===  OutDataTypeStr=boolean
  Compare To Zero3 : simulink/Logic and Bit Operations/Compare To Zero  relop=>  OutDataTypeStr=uint8
  Compare To Zero4 : simulink/Logic and Bit Operations/Compare To Zero  relop=>  OutDataTypeStr=uint8
  Constant : Constant  Value=P_VSM_TSR_SWS_speed_woDir
  Constant1 : Constant  Value=P_VSM_TSR_SWS_speed_withDir
  Constant2 : Constant  Value=P_VSM_TSR_SLW_SnvtySwitch
  Constant3 : Constant  Value=1.609  OutDataTypeStr=single
  Constant4 : Constant  Value=P_VSM_TSR_SteerWheelAngle
  Constant5 : Constant  OutDataTypeStr=Inherit: Inherit via back propagation
  Constant8 : Constant  Value=40  OutDataTypeStr=Inherit: Inherit via back propagation
  Product1 : Product  OutDataTypeStr=single
  Product3 : Product  OutDataTypeStr=single
  Relational Operator : RelationalOperator  Operator=>  OutDataTypeStr=boolean  RndMeth=Simplest
  Relational Operator1 : RelationalOperator  OutDataTypeStr=boolean  RndMeth=Simplest
  Saturation1 : Saturate  UpperLimit=10  LowerLimit=-10
  Saturation2 : Saturate  UpperLimit=5  LowerLimit=-5
  Saturation3 : Saturate  UpperLimit=5  LowerLimit=-5
  Saturation4 : Saturate  UpperLimit=10  LowerLimit=-10
  Sign : Signum
  Switch : Switch  Criteria=u2 > Threshold
  Switch1 : Switch  Criteria=u2 ~= 0
  Switch2 : Switch  Criteria=u2 ~= 0  OutDataTypeStr=single
  Switch3 : Switch  Criteria=u2 ~= 0  Threshold=1  OutDataTypeStr=single
  Switch4 : Switch  Criteria=u2 ~= 0  OutDataTypeStr=int8
  TSRResp : Outport
  TSRWarnResp : Outport  Port=2
  TSR_Snvty : Outport  Port=3  OutDataTypeStr=int8
  SLW_Snvty : Outport  Port=4  OutDataTypeStr=single
  SLW_Suppress : Outport  Port=5
  SLIF_Suppress : Outport  Port=6
  TS_Suppress : Outport  Port=7
  SLIF_LaneChange : Outport  Port=8  OutDataTypeStr=boolean
  wires:
  AND4/1 -> SLIF_Suppress/1  "VSM_TSR_SLIF_Suppress"
  Abs/1 -> Add/2
  VehYawRate/1 -> Abs/1, Sign/1
  Sign/1 -> Switch/2
  Compare To Zero/1 -> Switch/1
  RTurnLmpSwtSts/1 -> Compare To Zero1/1
  Switch1/1 -> Add/1
  Compare To Zero1/1 -> Switch/3
  Constant/1 -> Switch1/3
  Switch/1 -> Switch1/2
  Constant1/1 -> Switch1/1
  LTurnLmpSwtSts/1 -> Compare To Zero/1
  Add/1 -> Compare To Zero3/1  "SLIF_LaneChange"
  AND/1 -> SLW_Suppress/1  "VSM_TSR_SLW_Suppress"
  ISLActive_sts/1 -> AND/2
  Compare To Constant1/1 -> AND1/2
  Compare To Constant/1 -> AND1/1
  AND1/1 -> AND2/2  "SLW_EnableSpd_flag"
  AND5/1 -> AND2/3, TSRWarnResp/1
  AND2/1 -> AND/1  "SLW_EnableSpd_flag"
  Compare To Constant2/1 -> AND3/1
  AND3/1 -> AND4/2  "SLIF_EnableSpd_flag"
  Compare To Constant3/1 -> AND3/2
  VehSpd/1 -> [VehSpd], Compare To Constant3/1, Compare To Constant2/1
  TSRSwtReq/1 -> Compare To Zero2/1, AND2/1, AND4/1, AND5/1, TSRResp/1  "TSRSwtReq"
  TSRWarnSwtReq/1 -> AND5/2  "TSRWarnSwtReq"
  Compare To Zero2/1 -> TS_Suppress/1  "VSM_TSR_TS_Suppress"
  Compare To Zero3/1 -> AND6/1  "SLIF_Uturn"
  Constant2/1 -> Switch2/2
  Switch2/1 -> SLW_Snvty/1
  SteerWheelAngle/1 -> Relational Operator1/1, Relational Operator/1
  Constant4/1 -> Relational Operator/2
  Relational Operator/1 -> AND7/2
  AND6/1 -> SLIF_LaneChange/1  "SLIF_LaneChange"
  [VehSpd] -> Compare To Constant4/1
  Compare To Constant4/1 -> AND7/1
  AND7/1 -> AND6/2
  SPL_noSupp_Value/1 -> Compare To Constant1/1, Compare To Constant/1  "SPL_noSupp_Value"
  Switch3/1 -> Switch2/3  "SnvtyFactor"
  [IP_VehSpdUnit] -> Switch3/2
  Constant5/1 -> Product3/2
  TSR_SnvtySet/1 -> Saturation1/1, Saturation3/1, Switch2/1, Saturation4/1, Saturation2/1  "SLW_Snvty"
  Constant3/1 -> Product1/2
  Product1/1 -> Switch3/1  "SLW_Snvty"
  Product3/1 -> Switch3/3  "SLW_Snvty"
  Saturation3/1 -> Product1/1
  Saturation1/1 -> Product3/1
  Switch4/1 -> TSR_Snvty/1
  IP_VehSpdUnit/1 -> [IP_VehSpdUnit]
  [IP_VehSpdUnit] -> Switch4/2
  Saturation2/1 -> Switch4/1
  Saturation4/1 -> Switch4/3
  [VehSpd] -> Chart/1(Speed)
  Constant8/1 -> Relational Operator1/2
  Relational Operator1/1 -> Chart/2(temp)
  Chart/1(Turn_Flag) -> Compare To Zero4/1
  Compare To Zero4/1 -> AND6/3

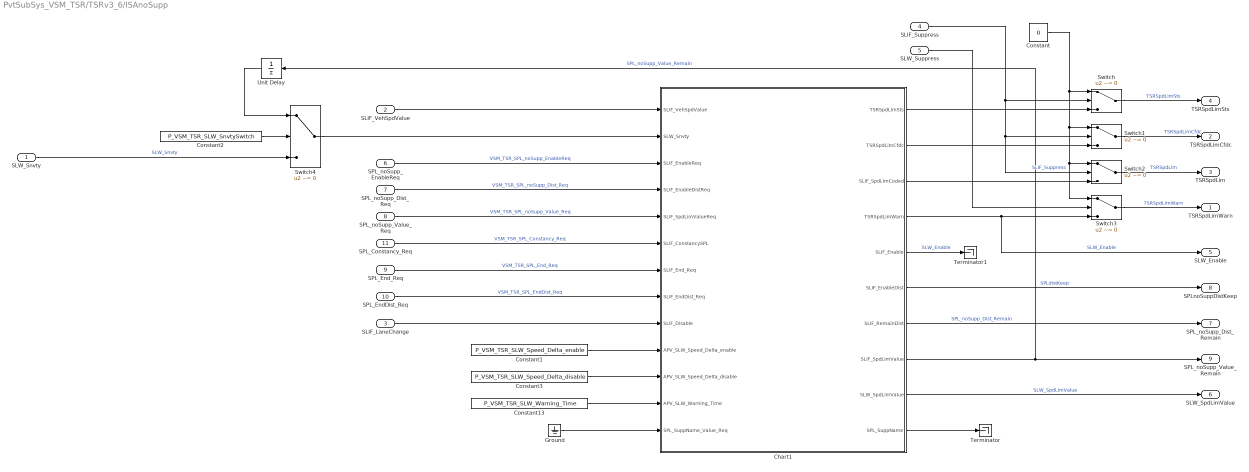
== system PvtSubSys_VSM_TSR/TSRv3_6/ISAnoSupp ==
  SLW_Snvty : Inport  OutDataTypeStr=single
  SLIF_VehSpdValue : Inport  Port=2  OutDataTypeStr=single
  SLIF_LaneChange : Inport  Port=3  OutDataTypeStr=boolean
  SLIF_Suppress : Inport  Port=4  OutDataTypeStr=boolean
  SLW_Suppress : Inport  Port=5
  SPL_noSupp_EnableReq : Inport  Port=6  OutDataTypeStr=boolean
  SPL_noSupp_Dist_Req : Inport  Port=7  OutDataTypeStr=single
  SPL_noSupp_Value_Req : Inport  Port=8  OutDataTypeStr=uint8
  SPL_End_Req : Inport  Port=9  OutDataTypeStr=boolean
  SPL_EndDist_Req : Inport  Port=10  OutDataTypeStr=single
  SPL_Constancy_Req : Inport  Port=11  OutDataTypeStr=uint8
  Chart1 : Stateflow chart  TreatAsAtomicUnit=on
  Constant : Constant  Value=0  OutDataTypeStr=Inherit: Inherit via back propagation
  Constant1 : Constant  Value=P_VSM_TSR_SLW_Speed_Delta_enable
  Constant13 : Constant  Value=P_VSM_TSR_SLW_Warning_Time
  Constant2 : Constant  Value=P_VSM_TSR_SLW_SnvtySwitch
  Constant3 : Constant  Value=P_VSM_TSR_SLW_Speed_Delta_disable
  Ground : Ground
  Switch{,1..3} (4 alike) : Switch  Criteria=u2 ~= 0
  Switch4 : Switch  Criteria=u2 ~= 0  OutDataTypeStr=single
  Terminator : Terminator
  Terminator1 : Terminator
  Unit Delay : UnitDelay  SampleTime=-1  HasFrameUpgradeWarning=on
  TSRSpdLimWarn : Outport
  TSRSpdLimCfdc : Outport  Port=2  OutDataTypeStr=uint8
  TSRSpdLim : Outport  Port=3
  TSRSpdLimSts : Outport  Port=4
  SLW_Enable : Outport  Port=5
  SLW_SpdLimValue : Outport  Port=6  OutDataTypeStr=uint8
  SPL_noSupp_Dist_Remain : Outport  Port=7  OutDataTypeStr=single
  SPLnoSuppDistKeep : Outport  Port=8
  SPL_noSupp_Value_Remain : Outport  Port=9
  wires:
  SLIF_Suppress/1 -> Switch/2, Switch1/2, Switch2/2  "SLIF_Suppress"
  SLIF_VehSpdValue/1 -> Chart1/1(SLIF_VehSpdValue)
  Chart1/4(TSRSpdLimWarn) -> SLW_Enable/1, Switch3/3  "SLW_Enable"
  Chart1/8(SLIF_SpdLimValue) -> Unit Delay/1, SPL_noSupp_Value_Remain/1  "SPL_noSupp_Value_Remain"
  Chart1/3(SLIF_SpdLimCoded) -> Switch2/3
  Chart1/6(SLIF_EnableDist) -> SPLnoSuppDistKeep/1  "SPLdistKeep"
  Chart1/7(SLIF_RemainDist) -> SPL_noSupp_Dist_Remain/1  "SPL_noSupp_Dist_Remain"
  Chart1/1(TSRSpdLimSts) -> Switch/3
  Chart1/9(SLW_SpdLimValue) -> SLW_SpdLimValue/1  "SLW_SpdLimValue"
  Chart1/2(TSRSpdLimCfdc) -> Switch1/3
  Switch/1 -> TSRSpdLimSts/1  "TSRSpdLimSts"
  Switch1/1 -> TSRSpdLimCfdc/1  "TSRSpdLimCfdc"
  Switch2/1 -> TSRSpdLim/1  "TSRSpdLim"
  Switch3/1 -> TSRSpdLimWarn/1  "TSRSpdLimWarn"
  SLW_Suppress/1 -> Switch3/2
  Constant/1 -> Switch3/1, Switch2/1, Switch1/1, Switch/1
  Constant1/1 -> Chart1/10(APV_SLW_Speed_Delta_enable)
  Constant3/1 -> Chart1/11(APV_SLW_Speed_Delta_disable)
  Constant13/1 -> Chart1/12(APV_SLW_Warning_Time)
  SPL_noSupp_EnableReq/1 -> Chart1/3(SLIF_EnableReq)  "VSM_TSR_SPL_noSupp_EnableReq"
  SPL_noSupp_Dist_Req/1 -> Chart1/4(SLIF_EnableDistReq)  "VSM_TSR_SPL_noSupp_Dist_Req"
  SPL_noSupp_Value_Req/1 -> Chart1/5(SLIF_SpdLimValueReq)  "VSM_TSR_SPL_noSupp_Value_Req"
  SPL_Constancy_Req/1 -> Chart1/6(SLIF_ConstancySPL)  "VSM_TSR_SPL_Constancy_Req"
  SPL_End_Req/1 -> Chart1/7(SLIF_End_Req)  "VSM_TSR_SPL_End_Req"
  SPL_EndDist_Req/1 -> Chart1/8(SLIF_EndDist_Req)  "VSM_TSR_SPL_EndDist_Req"
  SLIF_LaneChange/1 -> Chart1/9(SLIF_Disable)
  Ground/1 -> Chart1/13(SPL_SuppName_Value_Req)
  Chart1/10(SPL_SuppName) -> Terminator/1
  Constant2/1 -> Switch4/2
  SLW_Snvty/1 -> Switch4/3  "SLW_Snvty"
  Switch4/1 -> Chart1/2(SLW_Snvty)
  Unit Delay/1 -> Switch4/1
  Chart1/5(SLIF_Enable) -> Terminator1/1  "SLW_Enable"
